simulink model "digitalPLL_toneTrack"  (R2024b)
settings: Solver=FixedStepDiscrete  StartTime=0.0  StopTime=20  RelTol=1e-3
PostLoadFcn:
  | fs = 44100;
  | spf = 32;
  | 
  | fo = 60;
  | hilbf = designfilt('hilbertfir','FilterOrder',fo, ...
  |        'TransitionWidth',400,'SampleRate',fs);
  | hilb1 = hilbf.Numerator;
  | hilb2 = hilb1;
  | 
  | hilb1r = zeros(fo+1,1);
  | hilb2r = zeros(fo+1,1);
  | hilb1r(end) = 1;
  | hilb2r(end) = 1;
  | 
  | ncoclk = 1004;
libraries: dspsrcs4 x3, dspfdesign x1, dspsigops x1
settings Model: Creator=ftiong  LastModifiedBy=ftiong
settings SolverCC: AlgebraicLoopSolver=TrustRegion  AutoInsertRateTranBlk=on
settings DataIOCC: LimitDataPoints=on  SaveOutput=off  SignalLogging=off  SaveTime=off
settings OptimizationCC: ReuseModelBlockBuffer=off  LifeSpan=inf  SimCompilerOptimization=on
settings DebuggingCC: AlgebraicLoopMsg=error  SingleTaskRateTransMsg=error  UnconnectedInputMsg=warning  UnconnectedOutputMsg=warning  UnconnectedLineMsg=warning  AllowSymbolicDim=off  SubsystemReferenceDiagnosticForUnitTest=warning  SFUnexpectedBacktrackingDiag=warning  SFNoUnconditionalDefaultTransitionDiag=warning  SFExecutionAtInitializationDiag=none  ArithmeticOperatorsInVariantConditions=warning
settings ModelReferenceCC: EnableRefExpFcnMdlSchedulingChecks=on
settings SFSimCC: SimUseLocalCustomCode=off  CustomCodeUndefinedFunction=UseInterfaceOnly
settings RTWCC: RTWUseLocalCustomCode=off  GPUComputeCapability=3.5  LargeConstantGeneration=WriteOnlyDNNConstantsToDataFiles
settings CodeAppCC: StateflowObjectComments=on
settings GRTTargetCC: TargetLangStandard=C89/C90 (ANSI)
settings ConfigComp: CovMetricSettings=dw  CovSaveCumulativeToWorkspaceVar=on  CovSaveSingleToWorkspaceVar=on  CovExternalEMLEnable=off  CovSFcnEnable=off

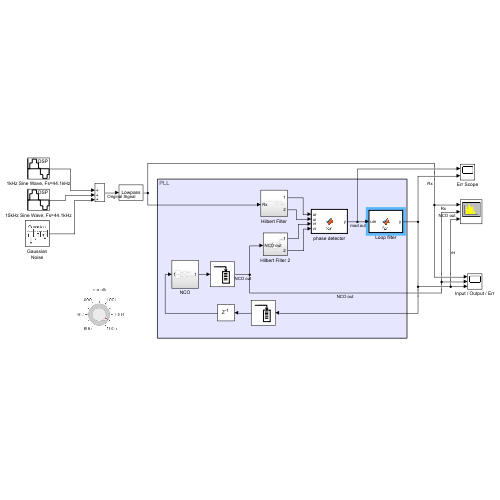
[thumbnail: Simulink's stored preview of the top-level diagram]
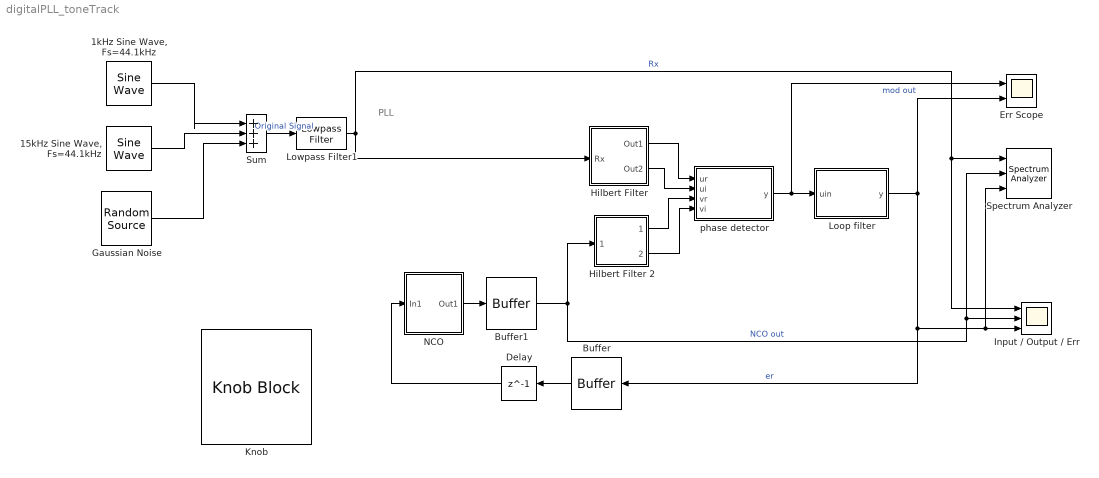
== system digitalPLL_toneTrack ==
  note: PLL
  "15kHz Sine Wave, Fs=44.1kHz" : dspsrcs4/Sine Wave  Amplitude=1  Frequency=15000  Phase=0  SampleMode=Discrete  OutComplex=Real  CompMethod=Trigonometric fcn  TableSize=Speed  SampleTime=1/fs  SamplesPerFrame=spf  ResetState=Restart at time zero  OutputFrames=off  dataType=double  wordLen=16  udDataType=sfix(16)  fracBitsMode=Best precision  numFracBits=15  OutDataTypeStr=double  LastOutDataTypeStr=double
  "1kHz Sine Wave, Fs=44.1kHz" : dspsrcs4/Sine Wave  Amplitude=1  Frequency=1000  Phase=0  SampleMode=Discrete  OutComplex=Real  CompMethod=Trigonometric fcn  TableSize=Speed  SampleTime=1/fs  SamplesPerFrame=spf  ResetState=Restart at time zero  OutputFrames=off  dataType=double  wordLen=16  udDataType=sfix(16)  fracBitsMode=Best precision  numFracBits=15  OutDataTypeStr=double  LastOutDataTypeStr=double
  Buffer : Buffer  N=1  OutputFrames=off
  Buffer1 : Buffer  N=spf  OutputFrames=off
  Delay : Delay  DelayLength=1
  Err Scope : Scope  NumInputPorts=2
  Gaussian Noise : dspsrcs4/Random Source  SrcType=Gaussian  MinVal=0  MaxVal=1  MeanVal=0  VarVal=.005  RepMode=Specify seed  rawSeed=1234567  IsInherit=off  SampTime=1/fs  SampFrame=spf  OutComplex=Real  DataType=double  SimulateUsing=Interpreted execution
  Hilbert Filter : Subsystem
  Hilbert Filter 2 : Subsystem
  Input / Output / Err : Scope  NumInputPorts=3
  Knob : KnobBlock  ScaleMin=995  ScaleMax=1005
  Loop filter : MATLAB Function  TreatAsAtomicUnit=on
  Lowpass Filter1 : dspfdesign/Lowpass Filter  FilterType=FIR  DesignForMinimumOrder=on  FilterOrder=50  PassbandFrequency=0.15  StopbandFrequency=0.3  PassbandRipple=0.1  StopbandAttenuation=80  SampleRateMode=Use normalized frequency (0 to 1)  SampleRate=44100  SimulateUsing=Interpreted execution  roundingMode=Floor  coeffsDataTypeStr=fixdt(1,16)
  NCO : Subsystem
  Spectrum Analyzer : SpectrumAnalyzer  NumInputPorts=3  WindowPosition=[320.000000,192.000000,641.000000,416.000000,]  Visible=on  ScopeFrameLocation=window  PlotAsTwoSidedSpectrum=off  YLimits=[-100.05984753,55.23010356]  ShowLegend=on
  Sum : Sum  Inputs=|+++
  phase detector : MATLAB Function  TreatAsAtomicUnit=on
  wires:
  "1kHz Sine Wave, Fs=44.1kHz"/1 -> Sum/1
  "15kHz Sine Wave, Fs=44.1kHz"/1 -> Sum/2
  Sum/1 -> Lowpass Filter1/1  "Original Signal"
  Gaussian Noise/1 -> Sum/3
  phase detector/1(y) -> Loop filter/1(uin), Err Scope/1  "mod out"
  Loop filter/1(y) -> Err Scope/2, Spectrum Analyzer/3, Input / Output / Err/3, Buffer/1  "er"
  Lowpass Filter1/1 -> Hilbert Filter/1(Rx), Input / Output / Err/1, Spectrum Analyzer/1  "Rx"
  Buffer/1 -> Delay/1
  Buffer1/1 -> Hilbert Filter 2/1(NCO out), Spectrum Analyzer/2, Input / Output / Err/2  "NCO out"
  Delay/1 -> NCO/1(In1)
  NCO/1(Out1) -> Buffer1/1
  Hilbert Filter/1(Out1) -> phase detector/1(ur)
  Hilbert Filter/2(Out2) -> phase detector/2(ui)
  Hilbert Filter 2/1(Out1) -> phase detector/3(vr)
  Hilbert Filter 2/2(Out2) -> phase detector/4(vi)

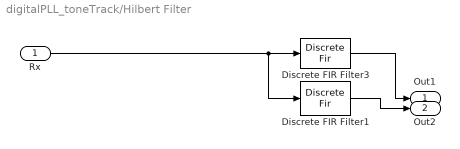
== system digitalPLL_toneTrack/Hilbert Filter ==
  Rx : Inport
  Discrete FIR Filter1 : DiscreteFir  Coefficients=hilb1  InputProcessing=Columns as channels (frame based)
  Discrete FIR Filter3 : DiscreteFir  Coefficients=hilb1r'  InputProcessing=Columns as channels (frame based)
  Out1 : Outport
  Out2 : Outport  Port=2
  wires:
  Rx/1 -> Discrete FIR Filter1/1, Discrete FIR Filter3/1
  Discrete FIR Filter3/1 -> Out1/1
  Discrete FIR Filter1/1 -> Out2/1

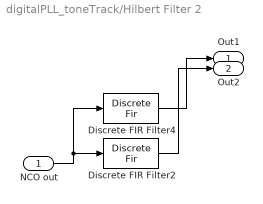
== system digitalPLL_toneTrack/Hilbert Filter 2 ==
  NCO out : Inport
  Discrete FIR Filter2 : DiscreteFir  Coefficients=hilb2  InputProcessing=Columns as channels (frame based)
  Discrete FIR Filter4 : DiscreteFir  Coefficients=hilb2r'  InputProcessing=Columns as channels (frame based)
  Out1 : Outport
  Out2 : Outport  Port=2
  wires:
  NCO out/1 -> Discrete FIR Filter4/1, Discrete FIR Filter2/1
  Discrete FIR Filter2/1 -> Out2/1
  Discrete FIR Filter4/1 -> Out1/1

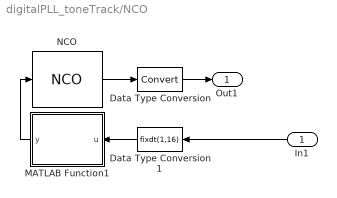
== system digitalPLL_toneTrack/NCO ==
  In1 : Inport
  Data Type Conversion : DataTypeConversion  SaturateOnIntegerOverflow=off  RndMeth=Floor
  Data Type Conversion1 : DataTypeConversion  OutMax=4  OutDataTypeStr=fixdt(1,16)  SaturateOnIntegerOverflow=off  RndMeth=Floor
  MATLAB Function1 : MATLAB Function  TreatAsAtomicUnit=on
  NCO : dspsigops/NCO  AccIncSrc=Input port  AccInc=2972  PhaseOffsetSrc=Specify via dialog  PhaseOffset=0  AccumWL=16  HasDither=on  DitherWL=4  PNgeneratorLength=19  HasPhaseQuantizer=on  TableDepth=12  HasOutputPhaseError=off  Formula=Sine  DataType=Binary point scaling  OutputWL=16  OutputFL=14  CompMethod=Table lookup (no interpolation)  SampleTime=1/44100  SamplesPerFrame=1  OutputFrames=off
  Out1 : Outport
  wires:
  In1/1 -> Data Type Conversion1/1
  NCO/1 -> Data Type Conversion/1
  MATLAB Function1/1(y) -> NCO/1
  Data Type Conversion1/1 -> MATLAB Function1/1(u)
  Data Type Conversion/1 -> Out1/1

== matlab function digitalPLL_toneTrack/NCO/MATLAB Function1 ==
  data: u input; y output; fs parameter; ncoclk parameter
function y = fcn(u, fs, ncoclk)

gain = 2;

constPhase = int16(ncoclk*(2^16)/fs);  % 1k = 1486
y = u*gain  + constPhase;

== matlab function digitalPLL_toneTrack/phase detector ==
  data: ur input; y output; ui input; vr input; vi input
function y = fcn(ur,ui,vr,vi)

eeps = 1e-7;

cu = complex(ur,ui);
cv = complex(vr,vi);

av = max(abs(cv),eeps);
au = max(abs(cu),eeps);


y = 2*(ur.*vi-ui.*vr).*(ur.*vr+ui.*vi);

== matlab function digitalPLL_toneTrack/Loop filter ==
  data: uin input; y output
function y = fcn(uin)

persistent memy; 

if isempty(memy)
    ss = length(uin);
    memy = zeros(ss,1);    
end



%% proportional integral loop filter 

t1 = 0.2;  
t2 = 0.1;
%T = 1/fs;

K2 = t2/t1;     
%K1 = T/t1;
K1 = (K2^2)/4;

yy = K1*uin + memy;
y = K2*uin + yy;
memy = yy;
